simulink model "sim_mot"  (R2020b)
settings: Solver=ode4  StartTime=0.0  StopTime=0.15  FixedStep=1e-5  RelTol=1e-3
values from neighbouring files (symbols this model uses):
  B1 = 6.64e-06    [sim_mot.mat]
  B2 = 1.476e-05    [sim_mot.mat]
  J1 = 3.43e-06    [sim_mot.mat]
  J2 = 6.48e-06    [sim_mot.mat]
  K1 = 0.0358    [sim_mot.mat]
  K2 = 0.0318    [sim_mot.mat]
  L1 = 0.00318    [sim_mot.mat]
  L2 = 0.00207    [sim_mot.mat]
  R1 = 7.27    [sim_mot.mat]
  R2 = 4.14    [sim_mot.mat]
settings Model: Creator=Erick  LastModifiedBy=Erick

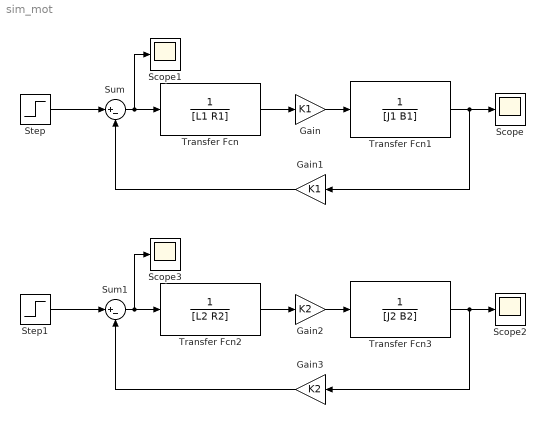
== system sim_mot ==
  Gain : Gain  Gain=K1
  Gain1 : Gain  Gain=K1
  Gain2 : Gain  Gain=K2
  Gain3 : Gain  Gain=K2
  Scope{,1..3} (4 alike) : Scope
  Step : Step  Time=0  After=24  SampleTime=0.2
  Step1 : Step  Time=0  After=24  SampleTime=0.2
  Sum : Sum  Inputs=|+-
  Sum1 : Sum  Inputs=|+-
  Transfer Fcn : TransferFcn  Denominator=[L1 R1]
  Transfer Fcn1 : TransferFcn  Denominator=[J1 B1]
  Transfer Fcn2 : TransferFcn  Denominator=[L2 R2]
  Transfer Fcn3 : TransferFcn  Denominator=[J2 B2]
  wires:
  Step/1 -> Sum/1
  Sum/1 -> Scope1/1, Transfer Fcn/1
  Transfer Fcn/1 -> Gain/1
  Gain/1 -> Transfer Fcn1/1
  Transfer Fcn1/1 -> Scope/1, Gain1/1
  Gain1/1 -> Sum/2
  Gain3/1 -> Sum1/2
  Sum1/1 -> Scope3/1, Transfer Fcn2/1
  Transfer Fcn3/1 -> Scope2/1, Gain3/1
  Transfer Fcn2/1 -> Gain2/1
  Step1/1 -> Sum1/1
  Gain2/1 -> Transfer Fcn3/1
